simulink library "Lib_EMTAT"  (R2023b)
settings: Solver=VariableStepAuto  StartTime=0.0  StopTime=10.0  RelTol=1e-3
undefined symbols (not defined in the file or in its folder): MWS
libraries: simulink x31, $bdroot x1
(part 1 of 4)
settings Model: Creator=sbianco1  LastModifiedBy=sbianco1
settings SolverCC: AlgebraicLoopSolver=TrustRegion
settings OptimizationCC: BlockReduction=off  DefaultParameterBehavior=Inlined  BufferReuse=off
settings DebuggingCC: UnconnectedInputMsg=warning  UnconnectedOutputMsg=warning  UnconnectedLineMsg=warning
settings ModelReferenceCC: EnableRefExpFcnMdlSchedulingChecks=on
settings RTWCC: DLArmComputeVersion=19.05

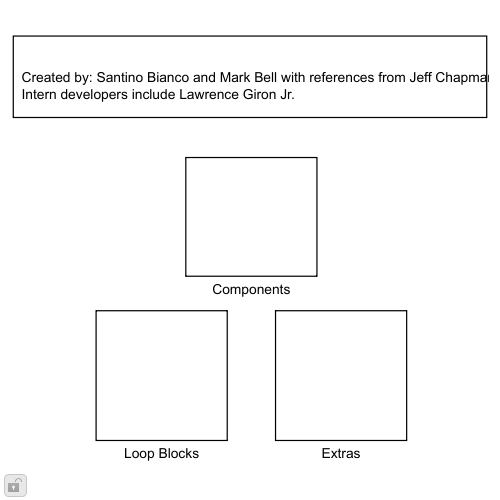
[thumbnail: Simulink's stored preview of the top-level diagram]
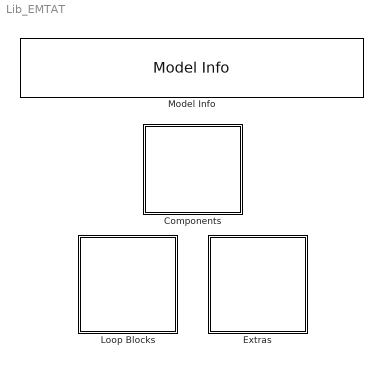
== system Lib_EMTAT ==
  Components : Subsystem
  Extras : Subsystem
  Loop Blocks : Subsystem
  Model Info : simulink/Model-Wide Utilities/Model Info  Frame=on  DisplayStringWithTags=|  HorizontalTextAlignment=Left  LeftAlignmentValue=0.02
      | Created by: Santino Bianco and Mark Bell with references from Jeff Chapman. 
      | Intern developers include Lawrence Giron Jr.

== system Lib_EMTAT/Components ==
  Physics-Based : Subsystem
  Power Flow : Subsystem

== system Lib_EMTAT/Extras ==
  Temperature with Cooling : Subsystem  mask(Component Temperature with Cooling (Ploss)){m=0, Cp=0, COP=0}
      mask prompts: m "m - Mass, lbm"; Cp "Cp - Specific Heat, Btu/(lbm-°F)"; COP "COP=(h*A_s) - Coefficient of Performance, Btu/(hr-°F)"
      mask help: This block calculates the temperature of a component based on the heat generated through power loss (Ploss) and the heat removed by a cooling system modeled as a generic heat exchanger. The block converts a power loss output in units of Watts (Ploss) from an electrical component to a temperature in units of °F (Temp) using the ambient temperature in units of °F (Tamb), and coolant temperature in units of °F (Tin_Cool) as inputs. A mass (m) in units of pound-mass, a specific heat (c_p) in units of Btu/(lbm-°F), and a coefficient of performance (COP) in units of Btu/(hr-°F) must be specified. The component temperature is integrated over time, and thus an initial heat (Q0) in units of Btu must be specified for the integrator block.
      settings: AttributesFormatString=Temperature with Cooling
      mask Help: web('Help_TemperaturewithCooling.html')
      mask DialogControl Container3 Prompt: Physical Parameters

== system Lib_EMTAT/Loop Blocks ==
  Outer Loop Integrator : Subsystem  mask(Outer Loop Integrator){Xo=0}
      mask prompts: Xo "Xo - Initial State Conditions"
      mask help: The Outer Loop Integrator takes in a vector of state variables and integrates each variable using a Continuous Integrator block.
      settings: AttributesFormatString=|
      | Outer Loop Integrator
      | Version: %<LibraryVersion>
      mask DialogControl fsfd Prompt: Parameters
  Outer Loop Time Step Delay : Subsystem  mask(Outer Loop Time Step Delay){Wo=0}
      mask prompts: Wo "Wo - Initial Conditions"
      mask help: The Outer Loop Time Step Delay block takes in a vector of variables and applies a one time step delay to each variable in the vector using a Unit Delay block.
      settings: AttributesFormatString=|
      | OuterLoop Time Step Delay
      | Version: %<LibraryVersion>
      mask DialogControl fsdf Prompt: Parameters

== system Lib_EMTAT/Components/Physics-Based ==

== system Lib_EMTAT/Components/Power Flow ==
  AC-AC Transformer (Efficiency Map) : Subsystem  mask(AC-AC Transformer (Efficiency Map)){X_C_VoltageAC1Vec_M=MWS.I1.Vdc, Y_C_CurrentAC2Vec_M=MWS.I1.Irms, T_C_EffArray_M=MWS.I1.Ploss', K=0.0503, FM=0}
      mask prompts: X_C_VoltageAC1Vec_M "X_C_VoltageAC1Vec_M - Primary AC Line to Neutral RMS Voltage Vector (X-axis)(nx1)"; Y_C_CurrentAC2Vec_M "Y_C_CurrentAC2Vec_M - Secondary RMS Line Current Vector (Y-axis)(mx1)"; T_C_EffArray_M "T_C_EffArray_M - Efficiency Table Values (Ploss = f(Irmsout, Vin)(nxm)"; K "K - Transformer Ratio"; FM "Mode:"
      mask help: This block models an AC/AC transofrmer. The power through the transformer is modified by a user-input efficiency table. The primary side is designated as 1. The secondary side is designated as 2.
      settings: AttributesFormatString=AC-AC Transformer (Efficiency Map)
      mask Help: web(['file:///' which('Help_ACACTransformer_EfficiencyMap.html')])
      mask DialogControl Control3 Prompt: Plot Efficiency Map
      mask DialogControl Control3 Callback:
      | % Plot efficiency map.
      | vals = get_param(gcb,'MaskValues');
      | X = str2num(cell2mat(vals(1)));
      | Y = str2num(cell2mat(vals(2)));
      | Z = str2num(cell2mat(vals(3)));
      | [X,Y] = meshgrid(X,Y);
      | figure('name',[get_param(gcb,'name') ' Efficiency Map'],'numbertitle','off')
      | contour(X,Y,Z,15);
      | xlabel('Voltage In, VDC')
      | ylabel('Line Current Out, A_{rms}')
      | title([get_param(gcb,'name') ' Efficiency Map'])
      | c = colorbar;
      | c.Label.String = 'Efficiency';
      mask DialogControl Container3 Prompt: Failure Modes
      mask DialogControl Control2 Prompt: 1 - Open Circuit, 2 - Degradation
  AC-AC Transformer (Power Loss Map) : Subsystem  mask(AC-AC Transformer (Power Loss Map)){X_C_VoltageAC1Vec_M=MWS.I1.Vdc, Y_C_CurrentAC2Vec_M=MWS.I1.Irms, T_C_PowLossArray_M=MWS.I1.Ploss', K=0.0503, FM=0, Plosslim=0}
      mask prompts: X_C_VoltageAC1Vec_M "X_C_VoltageAC1Vec_M - Primary AC Line to Neutral RMS Voltage Vector (X-axis)(nx1)"; Y_C_CurrentAC2Vec_M "Y_C_CurrentAC2Vec_M - Secondary RMS Line Current Vector (Y-axis)(mx1)"; T_C_PowLossArray_M "T_C_PowLossArray_M - Power Loss Table Values (Ploss = f(Irmsout, Vin)(nxm)"; K "K - Transformer Ratio"; FM "Mode:"; Plosslim "Plosslim - Power Loss Limit, W"
      mask help: This block models an AC/AC transofrmer. The power through the transformer is modified by a user-input power loss table. The primary side is designated as 1. The secondary side is designated as 2.
      settings: AttributesFormatString=AC-AC Transformer (Power Loss Map)
      mask Help: web(['file:///' which('Help_ACACTransformer_PowerLossMap.html')])
      mask DialogControl Control3 Prompt: Plot Power Loss Map
      mask DialogControl Control3 Callback:
      | % Plot efficiency map.
      | vals = get_param(gcb,'MaskValues');
      | X = str2num(cell2mat(vals(1)));
      | Y = str2num(cell2mat(vals(2)));
      | Z = str2num(cell2mat(vals(3)));
      | [X,Y] = meshgrid(X,Y);
      | figure('name',[get_param(gcb,'name') ' Power Loss Map'],'numbertitle','off')
      | contour(X,Y,Z,15);
      | xlabel('Voltage In, VDC')
      | ylabel('Line Current Out, A_{rms}')
      | title([get_param(gcb,'name') ' Power Loss Map'])
      | c = colorbar;
      | c.Label.String = 'Power Loss, W';
      mask DialogControl Container3 Prompt: Failure Modes
      mask DialogControl Control2 Prompt: 1 - Open Circuit, 2 - Degradation
  AC-DC Rectifier (Efficiency Map) : Subsystem  mask(AC - DC Rectifier (Efficiency Map)){X_C_VoltageInVec_M=[0 1000], Y_C_RMSCurrentOutVec_M=[0 1000], T_C_EffArray_M=ones(2), T_C_PFArray_M=ones(2), FM=0}
      mask prompts: X_C_VoltageInVec_M "X_C_VoltageInVec_M - DC Voltage Vector, V (m x 1)"; Y_C_RMSCurrentOutVec_M "Y_C_RMSCurrentOutVec_M - RMS Line Current Vector, Arms (p x 1)"; T_C_EffArray_M "T_C_EffArray_M - Efficiency Table Values, W (m x p)"; T_C_PFArray_M "T_C_PFArray_M - Power Factor Table Values, W (m x p)"; FM "Mode:"
      mask help: This block models an inverter/rectifier for use as a power source. The power through the inverter/rectifier is modified by a user-input efficiency and power factor tables.
      settings: AttributesFormatString=AC-DC Rectifier (Efficiency Map)
      mask Help: web(['file:///' which('Help_AC_DCRectifier_EfficiencyMap.html')])
      mask DialogControl Control2 Prompt: Plot Efficiency and Power Factor Maps
      mask DialogControl Control2 Callback:
      | % Plot efficiency map.
      | vals = get_param(gcb,'MaskValues');
      | X = str2num(cell2mat(vals(1)));
      | Y = str2num(cell2mat(vals(2)));
      | Z = str2num(cell2mat(vals(3)));
      | ZZ = str2num(cell2mat(vals(4)));
      | [X,Y] = meshgrid(X,Y);
      | figure('name',[get_param(gcb,'name') ' Efficiency and Power Factor Maps'],'numbertitle','off')
      | subplot(2,1,1)
      | contour(X,Y,Z,15);
      | xlabel('Voltage In, VDC')
      | ylabel('Line Current Out, A_{rms}')
      | title([get_param(gcb,'name') ' Efficiency Map'])
      | c = colorbar;
      | c.Label.String = 'Efficiency';
      | 
      | subplot(2,1,2)
      | contour(X,Y,ZZ,15);
      | xlabel('Voltage In, VDC')
      | ylabel('Line Current Out, A_{rms}')
      | title([get_param(gcb,'name') ' Power Factor Map'])
      | c = colorbar;
      | c.Label.String = 'Power Factor';
      mask DialogControl Container3 Prompt: Failure Modes
      mask DialogControl Control3 Prompt: 1 - Open Circuit, 2 - Efficiency Scalar
  AC-DC Rectifier (Power Loss Map) : Subsystem  mask(AC-DC Rectifier (Power Loss Map)){X_C_VoltageInVec_M=[0 1000], Y_C_RMSCurrentOutVec_M=[0 1000], T_C_PowLossArray_M=0*ones(2), T_C_PFArray_M=ones(2), FM=0, Plosslim=0}
      mask prompts: X_C_VoltageInVec_M "X_C_VoltageInVec_M - DC Voltage Vector, V (m x 1)"; Y_C_RMSCurrentOutVec_M "Y_C_RMSCurrentOutVec_M - RMS Line Current Vector, Arms (p x 1)"; T_C_PowLossArray_M "T_C_PowLossArray_M - Power Loss Table Values, W (m x p)"; T_C_PFArray_M "T_C_PFArray_M - Power Loss Table Values, W (m x p)"; FM "Mode:"; Plosslim "Plosslim - Power Loss Limit, W"
      mask help: This block models an inverter/rectifier for use as a power source. The power through the inverter/rectifier is modified by a user-input power loss and power factor tables.
      settings: AttributesFormatString=AC-DC Rectifier (Power Loss Map)
      mask Help: web(['file:///' which('Help_AC_DCRectifier_PowerLossMap.html')])
      mask DialogControl Control2 Prompt: Plot Power Loss and Power Factor Maps
      mask DialogControl Control2 Callback:
      | % Plot efficiency map.
      | vals = get_param(gcb,'MaskValues');
      | X = str2num(cell2mat(vals(1)));
      | Y = str2num(cell2mat(vals(2)));
      | Z = str2num(cell2mat(vals(3)));
      | ZZ = str2num(cell2mat(vals(4)));
      | [X,Y] = meshgrid(X,Y);
      | figure('name',[get_param(gcb,'name') ' Power Loss and Power Factor Maps'],'numbertitle','off')
      | subplot(2,1,1)
      | contour(X,Y,Z,15);
      | xlabel('Voltage In, VDC')
      | ylabel('Line Current Out, A_{rms}')
      | title([get_param(gcb,'name') ' Power Loss Map'])
      | c = colorbar;
      | c.Label.String = 'Power Loss, W';
      | 
      | subplot(2,1,2)
      | contour(X,Y,ZZ,15);
      | xlabel('Voltage In, VDC')
      | ylabel('Line Current Out, A_{rms}')
      | title([get_param(gcb,'name') ' Power Factor Map'])
      | c = colorbar;
      | c.Label.String = 'Power Factor';
      mask DialogControl Container3 Prompt: Failure Modes
      mask DialogControl Control3 Prompt: 1 - Open Circuit, 2 - Power Scalar
  Battery : Subsystem  mask(Generic Battery Model){ESR=0.005, Vcharge_vec=[3.60022000000000  3.47014090756723  3.40534522081438  3.36797345615108  3.34637300833001  3.33384164719904  3.32652442405484  3.32220404518678  3.31960513667983  3.31799408159663  3.31694886010866  3.31622666940565  3.31568778312557  3.31525175779256  3.31487224411964  3.31452249917241  3.31418705328483  3.31385691696240  3.31352682385014  3.31319364476023  3.31285547523761  3.31251111050485  3.31215974319668  3.31180078921639  3.31143378726315  3.31105834070993  3.31067408381608  3.31028066191027  3.30987771958033  3.30946489343758  3.30904180747880  3.30860806990567  3.30816327074273  3.30770697987113  3.30723874525401  3.30675809122011  3.30626451672401  3.30575749353022  3.30523646428523  3.30470084044935  3.30415000006513  3.30358328534007  3.30300000002157  3.30239940654061  3.30178072289873  3.30114311927020  3.30048571428812  3.29980757097933  3.29910769230854  3.29838501628717  3.29763841059637  3.29686666666691  3.29606849315088  3.29524250871097  3.29438723404271  3.29350108303264  3.29258235294130  3.29162921348325  3.29063969465657  3.28961167315181  3.28854285714290  3.28743076923078  3.28627272727272  3.28506582278477  3.28380689655166  3.28249251101312  3.28111891891878  3.27968202764960  3.27817735849035  3.27659999999974  3.27494455445513  3.27320507614176  3.27137499999957  3.26944705882304  3.26741318681262  3.26526440677901  3.26299069767368  3.26058083832252  3.25802222222128  3.25530063694161  3.25239999999879  3.24930204081497  3.24598591549143  3.24242773722455  3.23859999999805  3.23447086613954  3.23000327868604  3.22515384615104  3.21987142856824  3.21409532709918  3.20775294117234  3.20075670102620  3.19299999999457  3.18435172413165  3.17464878048051  3.16368571427719  3.15119999998996  3.13685074625673  3.12018709675987  3.10059999998259  3.07724615382467  3.04892340422834  3.01385714282250  2.96931351346777  2.91084999993737  2.83073333324329  2.71419999986125  2.52911764682123  2.18979999951267  1.36574285567986], Vdischarge_vec=[3.60022000000000  3.47014090756723  3.40534522081438  3.36797345615108  3.34637300833001  3.33384164719904  3.32652442405484  3.32220404518678  3.31960513667983  3.31799408159663  3.31694886010866  3.31622666940565  3.31568778312557  3.31525175779256  3.31487224411964  3.31452249917241  3.31418705328483  3.31385691696240  3.31352682385014  3.31319364476023  3.31285547523761  3.31251111050485  3.31215974319668  3.31180078921639  3.31143378726315  3.31105834070993  3.31067408381608  3.31028066191027  3.30987771958033  3.30946489343758  3.30904180747880  3.30860806990567  3.30816327074273  3.30770697987113  3.30723874525401  3.30675809122011  3.30626451672401  3.30575749353022  3.30523646428523  3.30470084044935  3.30415000006513  3.30358328534007  3.30300000002157  3.30239940654061  3.30178072289873  3.30114311927020  3.30048571428812  3.29980757097933  3.29910769230854  3.29838501628717  3.29763841059637  3.29686666666691  3.29606849315088  3.29524250871097  3.29438723404271  3.29350108303264  3.29258235294130  3.29162921348325  3.29063969465657  3.28961167315181  3.28854285714290  3.28743076923078  3.28627272727272  3.28506582278477  3.28380689655166  3.28249251101312  3.28111891891878  3.27968202764960  3.27817735849035  3.27659999999974  3.27494455445513  3.27320507614176  3.27137499999957  3.26944705882304  3.26741318681262  3.26526440677901  3.26299069767368  3.26058083832252  3.25802222222128  3.25530063694161  3.25239999999879  3.24930204081497  3.24598591549143  3.24242773722455  3.23859999999805  3.23447086613954  3.23000327868604  3.22515384615104  3.21987142856824  3.21409532709918  3.20775294117234  3.20075670102620  3.19299999999457  3.18435172413165  3.17464878048051  3.16368571427719  3.15119999998996  3.13685074625673  3.12018709675987  3.10059999998259  3.07724615382467  3.04892340422834  3.01385714282250  2.96931351346777  2.91084999993737  2.83073333324329  2.71419999986125  2.52911764682123  2.18979999951267  1.36574285567986], It_vec=[0  0.0209908023779841  0.0419816047559682  0.0629724071339524  0.0839632095119365  0.104954011889921  0.125944814267905  0.146935616645889  0.167926419023873  0.188917221401857  0.209908023779841  0.230898826157825  0.251889628535809  0.272880430913794  0.293871233291778  0.314862035669762  0.335852838047746  0.356843640425730  0.377834442803714  0.398825245181698  0.419816047559682  0.440806849937666  0.461797652315651  0.482788454693635  0.503779257071619  0.524770059449603  0.545760861827587  0.566751664205571  0.587742466583555  0.608733268961539  0.629724071339524  0.650714873717508  0.671705676095492  0.692696478473476  0.713687280851460  0.734678083229444  0.755668885607428  0.776659687985412  0.797650490363396  0.818641292741380  0.839632095119365  0.860622897497349  0.881613699875333  0.902604502253317  0.923595304631301  0.944586107009285  0.965576909387269  0.986567711765253  1.00755851414324  1.02854931652122  1.04954011889921  1.07053092127719  1.09152172365517  1.11251252603316  1.13350332841114  1.15449413078913  1.17548493316711  1.19647573554509  1.21746653792308  1.23845734030106  1.25944814267905  1.28043894505703  1.30142974743502  1.32242054981300  1.34341135219098  1.36440215456897  1.38539295694695  1.40638375932494  1.42737456170292  1.44836536408090  1.46935616645889  1.49034696883687  1.51133777121486  1.53232857359284  1.55331937597082  1.57431017834881  1.59530098072679  1.61629178310478  1.63728258548276  1.65827338786075  1.67926419023873  1.70025499261671  1.72124579499470  1.74223659737268  1.76322739975067  1.78421820212865  1.80520900450663  1.82619980688462  1.84719060926260  1.86818141164059  1.88917221401857  1.91016301639655  1.93115381877454  1.95214462115252  1.97313542353051  1.99412622590849  2.01511702828648  2.03610783066446  2.05709863304244  2.07808943542043  2.09908023779841  2.12007104017640  2.14106184255438  2.16205264493236  2.18304344731035  2.20403424968833  2.22502505206632  2.24601585444430  2.26700665682228  2.28799745920027]}
      mask prompts: ESR "Equivalent Series  Resistance - ESR (Ohm)"; Vcharge_vec "Battery Voltage Charge Curve (V)"; Vdischarge_vec "Battery Voltage Discharge Curve (V)"; It_vec "Capacity Table (Depth of Discharge) (Ah)"
      mask help: This is a block that models the voltage response of a generic battery based on the current demand. The block parameters are the internal resistance and the charge/discharge curves, which are defined as state of charge (SOC) vs. Voltage. Separate charge and discharge curves can be defined to allow for battery charge hysteresis.
      mask init:
      | BN = gcb;
      settings: AttributesFormatString=Battery
      mask Help: web(['file:///' which('Help_Battery.html')])
      mask DialogControl DescTextVar Prompt: Battery Model
  Cable : Subsystem  mask(Cable){R=0.2}
      mask prompts: R "R - Resistance, Ohm"
      mask help: This block models a cable with resistive effects.
      settings: AttributesFormatString=Cable
      mask Help: web(['file:///' which('Help_Cable.html')])
      mask DialogControl Container3 Prompt: Failure Modes
      mask DialogControl Control2 Prompt: Mode: Open Circuit
  Current Distribution : Subsystem  mask(Current Distribution){}
      settings: AttributesFormatString=Current Distribution
      mask Help: web(['file:///' which('Help_CurrentDistribution.html')])
  Current Junction : Subsystem  mask(Current Junction){Nb=1}
      mask prompts: Nb "Nb - # of branches"
      mask help: This block adds a vector of input currents (I).
      settings: AttributesFormatString=Current Junction
      mask Help: web(['file:///' which('Help_CurrentJunction.html')])
      mask DialogControl Control2 Prompt: Note: There is no limit to the number of multiplexed currents.
      mask DialogControl Container2 Prompt: Parameters
  DC-AC Inverter (Efficiency Map) : Subsystem  mask(DC-AC Inverter (Efficiency Map)){X_C_VoltageInVec_M=[0 1000], Y_C_RMSCurrentOutVec_M=[0 1000], T_C_EffArray_M=ones(2), T_C_PFArray_M=ones(2), K_e=0.0503, FM=0}
      mask prompts: X_C_VoltageInVec_M "X_C_VoltageInVec_M - DC Voltage Vector (X-axis)(nx1)"; Y_C_RMSCurrentOutVec_M "Y_C_RMSCurrentOutVec_M - RMS Line Current Vector (Y-axis)(mx1)"; T_C_EffArray_M "T_C_EffArray_M - Efficiency Table Values (Eff = f(Irmsout, Vin)(nxm)"; T_C_PFArray_M "T_C_PFArray_M - Power Factor Table Values (Eff = f(Irmsout, Vin)(nxm)"; K_e "K_e - Back EMF Constant, V_LL_peak/RPM"; FM "Mode:"
      mask help:
      | This block models an inverter/rectifier for use as a power sink. The power through the inverter/rectifier is modified by a user-input efficiency and power factor tables
      | .
      settings: AttributesFormatString=DC-AC Inverter (Efficiency Map)
      mask Help: web(['file:///' which('Help_DC_ACInverter_EfficiencyMap.html')])
      mask DialogControl Control3 Prompt: Plot Efficiency and Power Factor Maps
      mask DialogControl Control3 Callback:
      | % Plot efficiency map.
      | vals = get_param(gcb,'MaskValues');
      | X = str2num(cell2mat(vals(1)));
      | Y = str2num(cell2mat(vals(2)));
      | Z = str2num(cell2mat(vals(3)));
      | ZZ = str2num(cell2mat(vals(4)));
      | 
      | [X,Y] = meshgrid(X,Y);
      | figure('name',[get_param(gcb,'name') ' Efficiency and Power Factor Map'],'numbertitle','off')
      | subplot(2,1,1)
      | contour(X,Y,Z,15);
      | xlabel('Voltage In, VDC')
      | ylabel('Line Current Out, A_{rms}')
      | title([get_param(gcb,'name') ' Efficiency Map'])
      | c = colorbar;
      | c.Label.String = 'Efficiency';
      | 
      | subplot(2,1,2)
      | contour(X,Y,ZZ,15);
      | xlabel('Voltage In, VDC')
      | ylabel('Line Current Out, A_{rms}')
      | title([get_param(gcb,'name') ' Power Factor Map'])
      | c = colorbar;
      | c.Label.String = 'Power Factor';
      mask DialogControl Container3 Prompt: Failure Modes
      mask DialogControl Control2 Prompt: 1 - Open Circuit, 2 - Efficiency Scalar
  DC-AC Inverter (Power Loss Map) : Subsystem  mask(DC-AC Inverter (Power Loss Map)){X_C_VoltageInVec_M=[0 1000], Y_C_RMSCurrentOutVec_M=[0 1000], T_C_PowLossArray_M=zeros(2), T_C_PFArray_M=ones(2), K_e=0.0503, FM=0, Plosslim=0}
      mask prompts: X_C_VoltageInVec_M "X_C_VoltageInVec_M - DC Voltage Vector (X-axis)(nx1)"; Y_C_RMSCurrentOutVec_M "Y_C_RMSCurrentOutVec_M - RMS Line Current Vector (Y-axis)(mx1)"; T_C_PowLossArray_M "T_C_PowLossArray_M - Power Loss Table Values (Ploss = f(Irmsout, Vin)(nxm)"; T_C_PFArray_M "T_C_PFArray_M - Power Factor Table Values (Ploss = f(Irmsout, Vin)(nxm)"; K_e "K_e - Back EMF Constant, V_LL_peak/RPM"; FM "Mode:"; Plosslim "Plosslim - Power Loss Limit, W"
      mask help: This block models an inverter/rectifier for use as a power sink. The power through the inverter/rectifier is modified by a user-input power loss and power factor tables.
      settings: AttributesFormatString=DC-AC Inverter (Power Loss Map)
      mask Help: web(['file:///' which('Help_DC_ACInverter_PowerLossMap.html')])
      mask DialogControl Control3 Prompt: Plot Power Loss and Power Factor Maps
      mask DialogControl Control3 Callback:
      | % Plot efficiency map.
      | vals = get_param(gcb,'MaskValues');
      | X = str2num(cell2mat(vals(1)));
      | Y = str2num(cell2mat(vals(2)));
      | Z = str2num(cell2mat(vals(3)));
      | ZZ = str2num(cell2mat(vals(4)));
      | [X,Y] = meshgrid(X,Y);
      | figure('name',[get_param(gcb,'name') ' Power Loss and Power Factor Map'],'numbertitle','off')
      | subplot(2,1,1)
      | contour(X,Y,Z,15);
      | xlabel('Voltage In, VDC')
      | ylabel('Line Current Out, A_{rms}')
      | title([get_param(gcb,'name') ' Power Loss Map'])
      | c = colorbar;
      | c.Label.String = 'Power Loss, W';
      | 
      | subplot(2,1,2)
      | contour(X,Y,ZZ,15);
      | xlabel('Voltage In, VDC')
      | ylabel('Line Current Out, A_{rms}')
      | title([get_param(gcb,'name') ' Power Factor Map'])
      | c = colorbar;
      | c.Label.String = 'Power Factor';
      mask DialogControl Container3 Prompt: Failure Modes
      mask DialogControl Control2 Prompt: 1 - Open Circuit, 2 - Power Loss Scalar
  DC-DC Converter (Efficiency Map) (Regulate Output Voltage) : Subsystem  mask(DC-DC Converter (Efficiency Map) (Regulate Output Voltage)){X_Vin_VoltageVec_M=[0 100 1000 5000], Y_Iout_CurrentVec_M=[0 10 100 150], T_C_EffArray_M=0.98*ones(4,4), FM=0}
      mask prompts: X_Vin_VoltageVec_M "X_Vin_VoltageVec_M - Efficiency Table Voltage In Vector (X-axis)(nx1)"; Y_Iout_CurrentVec_M "Y_Iout_CurrentVec_M - Efficiency Table Current Out Vector (Y-axis)(mx1)"; T_C_EffArray_M "T_C_EffArray_M - Efficiency Table Values (Eff = f(i, V)(nxm)"; FM "Mode:"
      mask help: This block models the power flow through a DC-DC converter using a user specified efficiency table. The output voltage (Vout) can also be set using variable Vset.
      settings: AttributesFormatString=|
      | DC-DC Converter
      | (Efficiency Map)
      | (Regulate Output Voltage)
      mask Help: web(['file:///' which('Help_DCDCConverter_EfficiencyMap_RegulateOutputVoltage.html')])
      mask DialogControl Control3 Prompt: Plot Efficiency Map
      mask DialogControl Control3 Callback:
      | % Plot power loss map.
      | vals = get_param(gcb,'MaskValues');
      | X = str2num(cell2mat(vals(1)));
      | Y = str2num(cell2mat(vals(2)));
      | Z = str2num(cell2mat(vals(3)));
      | [X,Y] = meshgrid(X,Y);
      | figure('name',[get_param(gcb,'name') ' Efficiency Map'],'numbertitle','off')
      | contour(X,Y,Z,15);
      | xlabel('Voltage In, VDC')
      | ylabel('Current Out, ADC')
      | title([get_param(gcb,'name') ' Efficiency Map'])
      | c = colorbar;
      | c.Label.String = 'Efficiency';
      mask DialogControl Container3 Prompt: Failure Modes
      mask DialogControl Control2 Prompt: 1 - Open Circuit, 2 - Degradation
  DC-DC Converter (Efficiency Map) (Set Output Voltage) : Subsystem  mask(DC-DC Converter (Efficiency Map) (Set Output Voltage)){X_Vin_VoltageVec_M=[0 100 1000 5000], Y_Iout_CurrentVec_M=[0 10 100 150], T_C_EffArray_M=0.98*ones(4,4), FM=0}
      mask prompts: X_Vin_VoltageVec_M "X_Vin_VoltageVec_M - Efficiency Table Voltage In Vector, V (m x 1)"; Y_Iout_CurrentVec_M "Y_Iout_CurrentVec_M - Efficiency Table Current Out Vector, A (p x 1)"; T_C_EffArray_M "T_C_EffArray_M - Efficiency Table Values, W (m x p)"; FM "Mode:"
      mask help: This block models the power flow through a DC-DC converter using a user specified efficiency table. The output voltage (V_2) can be set using variable V*.
      settings: AttributesFormatString=|
      | DC-DC Converter
      | (Efficiency Map)
      | (Set Output Voltage)
      mask Help: web(['file:///' which('Help_DCDCConverter_EfficiencyMap_SetOutputVoltage.html')])
      mask DialogControl Control3 Prompt: Plot Efficiency Map
      mask DialogControl Control3 Callback:
      | % Plot power loss map.
      | vals = get_param(gcb,'MaskValues');
      | X = str2num(cell2mat(vals(1)));
      | Y = str2num(cell2mat(vals(2)));
      | Z = str2num(cell2mat(vals(3)));
      | [X,Y] = meshgrid(X,Y);
      | figure('name',[get_param(gcb,'name') ' Efficiency Map'],'numbertitle','off')
      | contour(X,Y,Z,15);
      | xlabel('Voltage In, VDC')
      | ylabel('Current Out, ADC')
      | title([get_param(gcb,'name') ' Efficiency Map'])
      | c = colorbar;
      | c.Label.String = 'Efficiency';
      mask DialogControl Container3 Prompt: Failure Modes
      mask DialogControl Control2 Prompt: 1 - Open Circuit, 2 - Degradation
  DC-DC Converter (Power Loss Map) (Regulate Output Voltage) : Subsystem  mask(DC-DC Converter (Power Loss Map) (Regulate Output Voltage)){X_Vin_VoltageVec_M=[0 100 1000 5000], Y_Iout_CurrentVec_M=[0 10 100 150], T_C_PlossArray_M=0.98*ones(4,4), FM=0, Plosslim=0}
      mask prompts: X_Vin_VoltageVec_M "X_Vin_VoltageVec_M - Efficiency Table Voltage In Vector (X-axis)(nx1)"; Y_Iout_CurrentVec_M "Y_Iout_CurrentVec_M - Efficiency Table Current Out Vector (Y-axis)(mx1)"; T_C_PlossArray_M "T_C_PlossArray_M - Power Loss Table Values (Eff = f(i, V)(nxm)"; FM "Mode:"; Plosslim "Plosslim - Power Loss Limit, W"
      mask help: This block models the power flow through a DC-DC converter using a user specified power loss table. The output voltage (Vout) can also be set using variable Vset.
      settings: AttributesFormatString=|
      | DC-DC Converter
      | (Power Loss Map)
      | (Regulate Output Voltage)
      mask Help: web(['file:///' which('Help_DCDCConverter_PowerLossMap_RegulateOutputVoltage.html')])
      mask DialogControl Control3 Prompt: Plot Power Loss Map
      mask DialogControl Control3 Callback:
      | % Plot power loss map.
      | vals = get_param(gcb,'MaskValues');
      | X = str2num(cell2mat(vals(1)));
      | Y = str2num(cell2mat(vals(2)));
      | Z = str2num(cell2mat(vals(3)));
      | [X,Y] = meshgrid(X,Y);
      | figure('name',[get_param(gcb,'name') ' Power Loss Map'],'numbertitle','off')
      | contour(X,Y,Z,15);
      | xlabel('Voltage In, VDC')
      | ylabel('Current Out, ADC')
      | title([get_param(gcb,'name') ' Power Loss Map'])
      | c = colorbar;
      | c.Label.String = 'Power loss, W';
      mask DialogControl Container3 Prompt: Failure Modes
      mask DialogControl Control2 Prompt: 1 - Open Circuit, 2 - Degradation
  DC-DC Converter (Power Loss Map) (Set Output Voltage) : Subsystem  mask(DC-DC Converter (Power Loss Map) (Set Output Voltage)){X_Vin_VoltageVec_M=[0 100 1000 5000], Y_Iout_CurrentVec_M=[0 10 100 150], T_C_PlossArray_M=0.98*ones(4,4), FM=0, Plosslim=0}
      mask prompts: X_Vin_VoltageVec_M "X_Vin_VoltageVec_M - Efficiency Table Voltage In Vector, V (m x 1)"; Y_Iout_CurrentVec_M "Y_Iout_CurrentVec_M - Efficiency Table Current Out Vector, A (p x 1)"; T_C_PlossArray_M "T_C_PlossArray_M - Power Loss Table Values, W (m x p)"; FM "Mode:"; Plosslim "Plosslim - Power Loss Limit, W"
      mask help: This block models the power flow through a DC-DC converter using a user specified power loss table. The output voltage (V_2) can be set using variable V*.
      settings: AttributesFormatString=|
      | DC-DC Converter
      | (Power Loss Map)
      | (Set Output Voltage)
      mask Help: web(['file:///' which('Help_DCDCConverter_PowerLossMap_SetOutputVoltage.html')])
      mask DialogControl Control3 Prompt: Plot Power Loss Map
      mask DialogControl Control3 Callback:
      | % Plot power loss map.
      | vals = get_param(gcb,'MaskValues');
      | X = str2num(cell2mat(vals(1)));
      | Y = str2num(cell2mat(vals(2)));
      | Z = str2num(cell2mat(vals(3)));
      | [X,Y] = meshgrid(X,Y);
      | figure('name',[get_param(gcb,'name') ' Power Loss Map'],'numbertitle','off')
      | contour(X,Y,Z,15);
      | xlabel('Voltage In, VDC')
      | ylabel('Current Out, ADC')
      | title([get_param(gcb,'name') ' Power Loss Map'])
      | c = colorbar;
      | c.Label.String = 'Power loss, W';
      mask DialogControl Container3 Prompt: Failure Modes
      mask DialogControl Control2 Prompt: 1 - Open Circuit, 2 - Degradation
  Electrical Bus : Subsystem  mask(Bus){C=6e-3, Nb=1}
      mask prompts: C "C - Capacitance, F"; Nb "Nb - # of branches"
      mask help: This block represents an electrical bus with capacitance effects.
      settings: AttributesFormatString=Electrical Bus
      mask Help: web(['file:///' which('Help_ElectricalBus.html')])
  Mechanical Shaft : Subsystem  mask(Mechanical Shaft){J=0.01, B=0.001}
      mask prompts: J "J - Inertia, lb-ft-s^2"; B "B - Damping, lb-ft-s"
      mask help: This block models a mechanical shaft with inertial and viscous damping effects.
      settings: AttributesFormatString=Mechanical Shaft
      mask Help: web(['file:///' which('Help_MechanicalShaft.html')])
      mask DialogControl Container3 Prompt: Failure Mode
      mask DialogControl Control2 Prompt: Mode: Shaft Break
  Power Supply (Set Voltage) : Subsystem  mask(Power Supply (Set Voltage)){Nb=0}
      mask prompts: Nb "Nb - # of branches"
      mask help: This block models a power supply that uses Vset to set, not regulate, the bus voltage based on a vector of current demands (Idmd).
      settings: AttributesFormatString=|
      | Power Supply
      | (Set Voltage)
      mask Help: web(['file:///' which('Help_PowerSupply_SetVoltage.html')])
      mask DialogControl Container2 Prompt: Parameters
  Resistive Load Bank : Subsystem  ClipboardFcn=|  mask(Resistive Load Bank){}
      | Active Resistor
      | Version: %<LibraryVersion>
      mask help: This block changes its resistance (R) based on a power command (Pset) to produce a current demand (Iin).
      settings: AttributesFormatString=Resistive Load Bank
      mask Help: web(['file:///' which('Help_ResistiveLoadBank.html')])
      mask DialogControl Container2 Prompt: Failure Modes
      mask DialogControl Control2 Prompt: Mode: Open Circuit
  Supercapacitor : Subsystem  mask(Supercapacitor){C=130, ESR=0.02, TSE=69, BlkNm=double(gcb)}
      mask prompts: C "C - Capacitance, F"; ESR "ESR - Equivilent Series Resistance, Ohm"; TSE "TSE - Max Stored Energy, W-h"; BlkNm "Block Name"
      mask help: This block models a capacitor with equivilent series resistive (ESR) effects.
      mask init:
      | BN = gcb;
      settings: AttributesFormatString=Supercapacitor
      mask Help: web(['file:///' which('Help_Supercapacitor.html')])
  Three Phase Electric Machine (Sink) : Subsystem  mask(Three Phase Electric Machine (Sink)){X_C_SpeedVec_M=[0 8000], Y_C_TorqueVec_M=[0 300], T_C_EffArray_M=[0.97 0.95; 0.93 0.94], T_C_PFArray_M=[1 1;1 1], FM=0}
      mask prompts: X_C_SpeedVec_M "X_C_SpeedVec_M - Efficiency Table Speed Vector (nx1)"; Y_C_TorqueVec_M "Y_C_TorqueVec_M - Efficiency Table Torque Vector (mx1)"; T_C_EffArray_M "T_C_EffArray_M - Efficiency Table Values (nxm)"; T_C_PFArray_M "T_C_PFArray_M - Power Factor Table Values (nxm)"; FM "Mode:"
      mask help: This block models an three phase motor/generator for use as a power sink. The power through the motor/generator is modified by a user-input efficiency and power factor tables.
      settings: AttributesFormatString=|
      | Three Phase Electric Machine
      | (Sink)
      mask Help: web(['file:///' which('Help_ThreePhaseElectricMachineSink.html')])
      mask DialogControl Container2 Prompt: Parameters
      mask DialogControl Plot Prompt: Plot Efficiency and Power Factor Maps
      mask DialogControl Plot Callback:
      | % Plot efficiency map.
      | vals = get_param(gcb,'MaskValues');
      | X = str2num(cell2mat(vals(1)));
      | Y = str2num(cell2mat(vals(2)));
      | Z = str2num(cell2mat(vals(3)));
      | ZZ = str2num(cell2mat(vals(4)));
      | [X,Y] = meshgrid(X,Y);
      | 
      | figure('name',[get_param(gcb,'name') ' Efficiency and Power Factor Map'],'numbertitle','off')
      | subplot(2,1,1)
      | contour(X,Y,Z,15);
      | xlabel('Speed, RPM')
      | ylabel('Torque, lbf-ft')
      | title([get_param(gcb,'name') ' Efficiency Map'])
      | c = colorbar;
      | c.Label.String = 'Efficiency';
      | 
      | subplot(2,1,2)
      | contour(X,Y,ZZ,15);
      | xlabel('Speed, RPM')
      | ylabel('Torque, lbf-ft')
      | title([get_param(gcb,'name') ' Power Factor Map'])
      | c = colorbar;
      | c.Label.String = 'Power Factor';
      mask DialogControl Container3 Prompt: Failure Modes
      mask DialogControl Control3 Prompt: 1 - Open Circuit, 2 - Efficiency Scaling
  Three Phase Electric Machine (Source) : Subsystem  mask(Three Phase Electric Machine (Source)){X_C_SpeedVec_M=[0 10000], Y_C_TorqueVec_M=[0 500], T_C_EffArray_M=0.9*ones(2), T_C_PFArray_M=[1,1;1,1], Ke=0.05, FM=0}
      mask prompts: X_C_SpeedVec_M "X_C_SpeedVec_M - Efficiency Table Speed Vector (X-axis)(nx1)"; Y_C_TorqueVec_M "Y_C_TorqueVec_M - Efficiency Table Torque Vector (Y-axis)(mx1)"; T_C_EffArray_M "T_C_EffArray_M - Efficiency Table Values (nxm)"; T_C_PFArray_M "T_C_PFArray_M - Power Fector Table Values (nxm)"; Ke "Ke - Back EMF Constant, V_LL_peak/RPM"; FM "Mode:"
      mask help: This block models an motor/generator for use as a power source. The power through the motor/generator is modified by a user-input efficiency and power factor tables.
      settings: AttributesFormatString=|
      | Three Phase Electric Machine
      | (Source)
      mask Help: web(['file:///' which('Help_ThreePhaseElectricMachineSource.html')])
      mask DialogControl Control2 Prompt: Plot Efficiency and Power Loss Maps
      mask DialogControl Control2 Callback:
      | % Plot efficiency map.
      | vals = get_param(gcb,'MaskValues');
      | X = str2num(cell2mat(vals(1)));
      | Y = str2num(cell2mat(vals(2)));
      | Z = str2num(cell2mat(vals(3)));
      | ZZ = str2num(cell2mat(vals(4)));
      | [X,Y] = meshgrid(X,Y);
      | 
      | figure('name',[get_param(gcb,'name') ' Efficiency and Power Factor Map'],'numbertitle','off')
      | subplot(2,1,1)
      | contour(X,Y,Z,15);
      | xlabel('Speed, RPM')
      | ylabel('Torque, lbf-ft')
      | title([get_param(gcb,'name') ' Efficiency Map'])
      | c = colorbar;
      | c.Label.String = 'Efficiency';
      | 
      | subplot(2,1,2)
      | contour(X,Y,ZZ,15);
      | xlabel('Speed, RPM')
      | ylabel('Torque, lbf-ft')
      | title([get_param(gcb,'name') ' Power Factor Map'])
      | c = colorbar;
      | c.Label.String = 'Power Factor';
      mask DialogControl Container3 Prompt: Failure Modes
      mask DialogControl Control3 Prompt: 1 - Open Circuit, 2 - Efficiency Scalar

== system Lib_EMTAT/Extras/Temperature with Cooling ==
  "Ploss, W" : Inport
  "Tamb, degF" : Inport  Port=2
  "Tcool, degF" : Inport  Port=3
  "T(t-1), degF" : Inport  Port=4
  "Q, J" : Inport  Port=5
  BTU/hr to Watts : Gain  Gain=0.29307
  Coefficient of Performance (Btu/(hr-°F)) : Constant  Value=COP
  Divide : Product  Inputs=*//
  Joules to BTU : Gain  Gain=0.000947817
  Mass (lbm) : Constant  Value=m
  Multiply1 : Product  Inputs=**
  Specific Heat (Btu/(lbm-°F)) : Constant  Value=Cp
  Subtract : Sum  Inputs=-+
  Subtract2 : Sum  Inputs=+-
  Sum : Sum  Inputs=|++
  "T, degF" : Outport
  "T(t), degF" : Outport  Port=2
  "Qdot, W" : Outport  Port=3
  wires:
  "Tamb, degF"/1 -> Sum/2
  Joules to BTU/1 -> Divide/1
  Specific Heat (Btu/(lbm-°F))/1 -> Divide/3
  Coefficient of Performance (Btu/(hr-°F))/1 -> Multiply1/2
  "Q, J"/1 -> Joules to BTU/1
  "Tcool, degF"/1 -> Subtract2/2
  Subtract2/1 -> Multiply1/1
  Sum/1 -> "T(t), degF"/1, "T, degF"/1
  "T(t-1), degF"/1 -> Subtract2/1
  "Ploss, W"/1 -> Subtract/2
  Mass (lbm)/1 -> Divide/2
  Divide/1 -> Sum/1
  Subtract/1 -> "Qdot, W"/1
  Multiply1/1 -> BTU/hr to Watts/1
  BTU/hr to Watts/1 -> Subtract/1

== system Lib_EMTAT/Loop Blocks/Outer Loop Integrator ==
  Xdot : Inport
  Constant : Constant  Value=Xo
  Integrator : Integrator  InitialConditionSource=external
  X : Outport
  wires:
  Integrator/1 -> X/1
  Xdot/1 -> Integrator/1
  Constant/1 -> Integrator/2

== system Lib_EMTAT/Loop Blocks/Outer Loop Time Step Delay ==
  W(t) : Inport
  Unit Delay : UnitDelay  InitialCondition=Wo  SampleTime=-1  HasFrameUpgradeWarning=on
  W(t-1) : Outport
  wires:
  W(t)/1 -> Unit Delay/1
  Unit Delay/1 -> W(t-1)/1

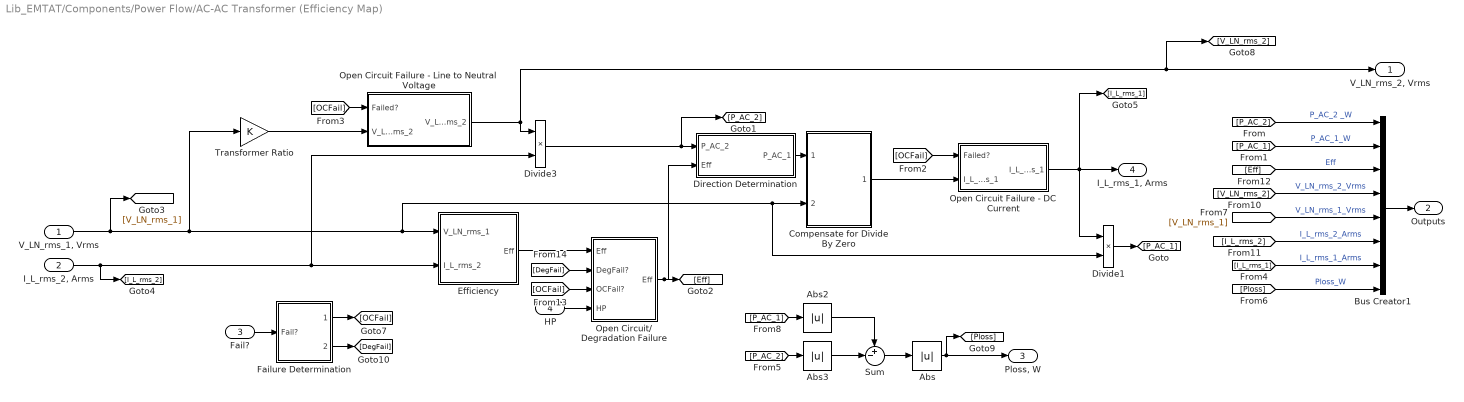
== system Lib_EMTAT/Components/Power Flow/AC-AC Transformer (Efficiency Map) ==
  "V_LN_rms_1, Vrms" : Inport
  "I_L_rms_2, Arms" : Inport  Port=2
  Fail? : Inport  Port=3
  HP : Inport  Port=4
  Abs : Abs  SaturateOnIntegerOverflow=off
  Abs2 : Abs  SaturateOnIntegerOverflow=off
  Abs3 : Abs  SaturateOnIntegerOverflow=off
  Bus Creator1 : BusCreator  Inputs=8
  Compensate for Divide By Zero : Subsystem
  Direction Determination : Subsystem
  Divide1 : Product  Inputs=**
  Divide3 : Product  Inputs=**
  Efficiency : Subsystem
  Failure Determination : Subsystem
  Open Circuit Failure - DC Current : Subsystem
  Open Circuit Failure - Line to Neutral Voltage : Subsystem
  Open Circuit/ Degradation Failure : Subsystem
  Sum : Sum  Inputs=+-|
  Transformer Ratio : Gain  Gain=K
  "V_LN_rms_2, Vrms" : Outport
  Outputs : Outport  Port=2
  "Ploss, W" : Outport  Port=3
  "I_L_rms_1, Arms" : Outport  Port=4
  wires:
  [DegFail] -> Open Circuit/ Degradation Failure/2(DegFail?)
  [OCFail] -> Open Circuit/ Degradation Failure/3(OCFail?)
  HP/1 -> Open Circuit/ Degradation Failure/4(HP)
  Fail?/1 -> Failure Determination/1(Fail?)
  Failure Determination/1(OCFail) -> [OCFail]
  Failure Determination/2(DegFail) -> [DegFail]
  Efficiency/1(Eff) -> Open Circuit/ Degradation Failure/1(Eff)
  Open Circuit Failure - Line to Neutral Voltage/1("V_LN_rms_2 ") -> Divide3/1, [V_LN_rms_2], "V_LN_rms_2, Vrms"/1
  [OCFail] -> Open Circuit Failure - Line to Neutral Voltage/1(Failed?)
  Transformer Ratio/1 -> Open Circuit Failure - Line to Neutral Voltage/2(V_LN_rms_2)
  [OCFail] -> Open Circuit Failure - DC Current/1(Failed?)
  [Eff] -> Bus Creator1/3  "Eff"
  [I_L_rms_2] -> Bus Creator1/6  "I_L_rms_2_Arms"
  [Ploss] -> Bus Creator1/8  "Ploss_W"
  [I_L_rms_1] -> Bus Creator1/7  "I_L_rms_1_Arms"
  [V_LN_rms_1] -> Bus Creator1/5  "V_LN_rms_1_Vrms"
  [V_LN_rms_2] -> Bus Creator1/4  "V_LN_rms_2_Vrms"
  "I_L_rms_2, Arms"/1 -> [I_L_rms_2], Divide3/2, Efficiency/2(I_L_rms_2)
  Divide3/1 -> Direction Determination/1(P_AC_2), [P_AC_2]
  Open Circuit Failure - DC Current/1("I_L_rms_1 ") -> [I_L_rms_1], "I_L_rms_1, Arms"/1, Divide1/1
  Open Circuit/ Degradation Failure/1("Eff ") -> Direction Determination/2(Eff), [Eff]
  [P_AC_1] -> Bus Creator1/2  "P_AC_1_W"
  [P_AC_2] -> Bus Creator1/1  "P_AC_2 _W"
  Bus Creator1/1 -> Outputs/1
  Direction Determination/1(P_AC_1) -> Compensate for Divide By Zero/1(P_AC_1)
  Divide1/1 -> [P_AC_1]
  "V_LN_rms_1, Vrms"/1 -> Transformer Ratio/1, Divide1/2, Compensate for Divide By Zero/2(V_LN_rms_1), Efficiency/1(V_LN_rms_1), [V_LN_rms_1]
  Compensate for Divide By Zero/1(I_L_rms_1) -> Open Circuit Failure - DC Current/2(I_L_rms_1)
  Abs2/1 -> Sum/1
  Sum/1 -> Abs/1
  [P_AC_1] -> Abs2/1
  Abs3/1 -> Sum/2
  Abs/1 -> "Ploss, W"/1, [Ploss]
  [P_AC_2] -> Abs3/1

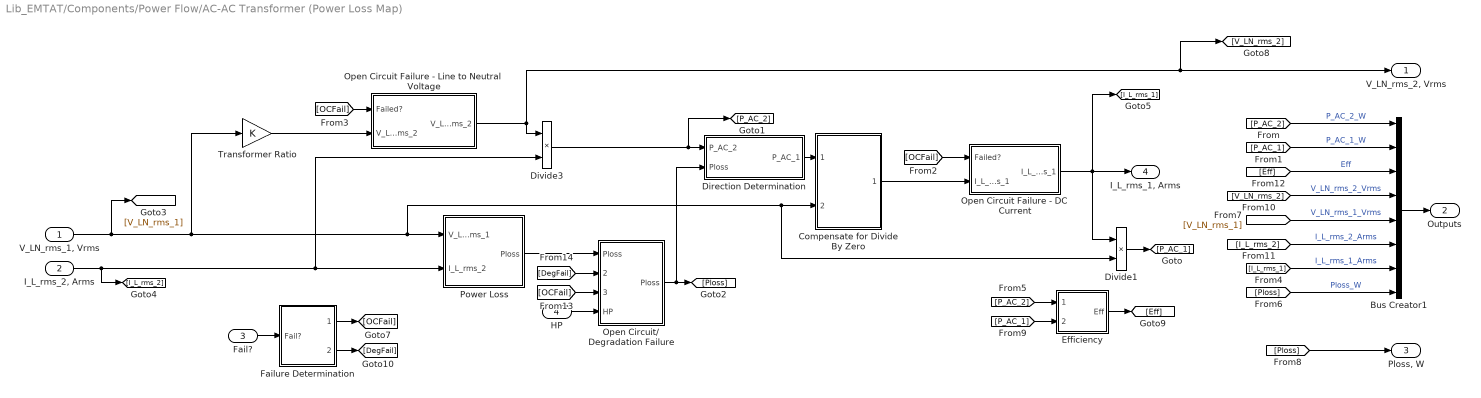
== system Lib_EMTAT/Components/Power Flow/AC-AC Transformer (Power Loss Map) ==
  "V_LN_rms_1, Vrms" : Inport
  "I_L_rms_2, Arms" : Inport  Port=2
  Fail? : Inport  Port=3
  HP : Inport  Port=4
  Bus Creator1 : BusCreator  Inputs=8
  Compensate for Divide By Zero : Subsystem
  Direction Determination : Subsystem
  Divide1 : Product  Inputs=**
  Divide3 : Product  Inputs=**
  Efficiency : Subsystem
  Failure Determination : Subsystem
  Open Circuit Failure - DC Current : Subsystem
  Open Circuit Failure - Line to Neutral Voltage : Subsystem
  Open Circuit/ Degradation Failure : Subsystem
  Power Loss : Subsystem
  Transformer Ratio : Gain  Gain=K
  "V_LN_rms_2, Vrms" : Outport
  Outputs : Outport  Port=2
  "Ploss, W" : Outport  Port=3
  "I_L_rms_1, Arms" : Outport  Port=4
  wires:
  Compensate for Divide By Zero/1(I_L_rms_1) -> Open Circuit Failure - DC Current/2(I_L_rms_1)
  "V_LN_rms_1, Vrms"/1 -> [V_LN_rms_1], Power Loss/1(V_LN_rms_1), Compensate for Divide By Zero/2(V_LN_rms_1), Divide1/2, Transformer Ratio/1
  Divide1/1 -> [P_AC_1]
  Direction Determination/1(P_AC_1) -> Compensate for Divide By Zero/1(P_AC_1)
  Bus Creator1/1 -> Outputs/1
  [P_AC_2] -> Bus Creator1/1  "P_AC_2_W"
  [P_AC_1] -> Bus Creator1/2  "P_AC_1_W"
  Open Circuit/ Degradation Failure/1("Ploss ") -> Direction Determination/2(Ploss), [Ploss]
  Open Circuit Failure - DC Current/1("I_L_rms_1 ") -> Divide1/1, "I_L_rms_1, Arms"/1, [I_L_rms_1]
  Divide3/1 -> Direction Determination/1(P_AC_2), [P_AC_2]
  [Ploss] -> "Ploss, W"/1
  "I_L_rms_2, Arms"/1 -> Power Loss/2(I_L_rms_2), Divide3/2, [I_L_rms_2]
  [V_LN_rms_2] -> Bus Creator1/4  "V_LN_rms_2_Vrms"
  [V_LN_rms_1] -> Bus Creator1/5  "V_LN_rms_1_Vrms"
  [I_L_rms_1] -> Bus Creator1/7  "I_L_rms_1_Arms"
  [Ploss] -> Bus Creator1/8  "Ploss_W"
  [I_L_rms_2] -> Bus Creator1/6  "I_L_rms_2_Arms"
  [P_AC_1] -> Efficiency/2(P_AC_1)
  [P_AC_2] -> Efficiency/1(P_AC_2)
  Efficiency/1(Eff) -> [Eff]
  [Eff] -> Bus Creator1/3  "Eff"
  [OCFail] -> Open Circuit Failure - DC Current/1(Failed?)
  Transformer Ratio/1 -> Open Circuit Failure - Line to Neutral Voltage/2(V_LN_rms_2)
  [OCFail] -> Open Circuit Failure - Line to Neutral Voltage/1(Failed?)
  Open Circuit Failure - Line to Neutral Voltage/1("V_LN_rms_2 ") -> "V_LN_rms_2, Vrms"/1, [V_LN_rms_2], Divide3/1
  Power Loss/1(Ploss) -> Open Circuit/ Degradation Failure/1(Ploss)
  Failure Determination/2(DegFail) -> [DegFail]
  Failure Determination/1(OCFail) -> [OCFail]
  Fail?/1 -> Failure Determination/1(Fail?)
  HP/1 -> Open Circuit/ Degradation Failure/4(HP)
  [OCFail] -> Open Circuit/ Degradation Failure/3(OCFail?)
  [DegFail] -> Open Circuit/ Degradation Failure/2(DegFail?)

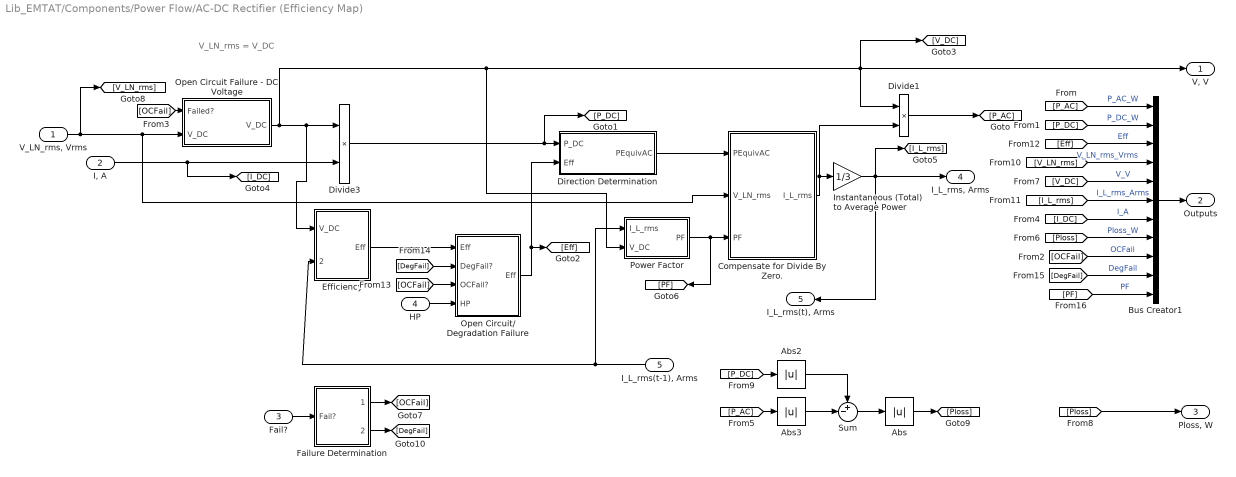
== system Lib_EMTAT/Components/Power Flow/AC-DC Rectifier (Efficiency Map) ==
  note: V_LN_rms = V_DC
  "V_LN_rms, Vrms" : Inport
  "I, A" : Inport  Port=2
  Fail? : Inport  Port=3
  HP : Inport  Port=4
  "I_L_rms(t-1), Arms" : Inport  Port=5
  Abs : Abs  SaturateOnIntegerOverflow=off
  Abs2 : Abs  SaturateOnIntegerOverflow=off
  Abs3 : Abs  SaturateOnIntegerOverflow=off
  Bus Creator1 : BusCreator  Inputs=11
  Compensate for Divide By Zero. : Subsystem
  Direction Determination : Subsystem
  Divide1 : Product  Inputs=**
  Divide3 : Product  Inputs=**
  Efficiency : Subsystem
  Failure Determination : Subsystem
  Instantaneous (Total) to Average Power : Gain  Gain=1/3
  Open Circuit Failure - DC Voltage : Subsystem
  Open Circuit/ Degradation Failure : Subsystem
  Power Factor : Subsystem
  Sum : Sum  Inputs=+-|
  "V, V " : Outport
  Outputs : Outport  Port=2
  "Ploss, W" : Outport  Port=3
  "I_L_rms, Arms" : Outport  Port=4
  "I_L_rms(t), Arms" : Outport  Port=5
  wires:
  Divide1/1 -> [P_AC]
  "I, A"/1 -> [I_DC], Divide3/2
  Compensate for Divide By Zero./1(I_L_rms) -> Divide1/2, Instantaneous (Total) to Average Power/1
  [Eff] -> Bus Creator1/3  "Eff"
  [I_L_rms] -> Bus Creator1/6  "I_L_rms_Arms"
  [Ploss] -> Bus Creator1/8  "Ploss_W"
  [I_DC] -> Bus Creator1/7  "I_A"
  [V_DC] -> Bus Creator1/5  "V_V"
  [V_LN_rms] -> Bus Creator1/4  "V_LN_rms_Vrms"
  [Ploss] -> "Ploss, W"/1
  Divide3/1 -> Direction Determination/1(P_DC), [P_DC]
  Open Circuit/ Degradation Failure/1("Eff ") -> Direction Determination/2(Eff), [Eff]
  [P_DC] -> Bus Creator1/2  "P_DC_W"
  [P_AC] -> Bus Creator1/1  "P_AC_W"
  Bus Creator1/1 -> Outputs/1
  Direction Determination/1(PEquivAC) -> Compensate for Divide By Zero./1(PEquivAC)
  "I_L_rms(t-1), Arms"/1 -> Efficiency/2(I_L_rms), Power Factor/1(I_L_rms)
  Instantaneous (Total) to Average Power/1 -> [I_L_rms], "I_L_rms(t), Arms"/1, "I_L_rms, Arms"/1
  [OCFail] -> Open Circuit Failure - DC Voltage/1(Failed?)
  "V_LN_rms, Vrms"/1 -> [V_LN_rms], Compensate for Divide By Zero./2(V_LN_rms), Open Circuit Failure - DC Voltage/2(V_DC)
  [OCFail] -> Open Circuit/ Degradation Failure/3(OCFail?)
  [DegFail] -> Open Circuit/ Degradation Failure/2(DegFail?)
  HP/1 -> Open Circuit/ Degradation Failure/4(HP)
  Efficiency/1(Eff) -> Open Circuit/ Degradation Failure/1(Eff)
  Fail?/1 -> Failure Determination/1(Fail?)
  Failure Determination/2(DegFail) -> [DegFail]
  Failure Determination/1(OCFail) -> [OCFail]
  Open Circuit Failure - DC Voltage/1("V_DC ") -> Efficiency/1(V_DC), Divide3/1, "V, V "/1, Divide1/1, [V_DC], Power Factor/2(V_DC)
  [P_AC] -> Abs3/1
  Abs3/1 -> Sum/2
  [P_DC] -> Abs2/1
  Sum/1 -> Abs/1
  Abs2/1 -> Sum/1
  Abs/1 -> [Ploss]
  Power Factor/1(PF) -> [PF], Compensate for Divide By Zero./3(PF)
  [OCFail] -> Bus Creator1/9  "OCFail"
  [DegFail] -> Bus Creator1/10  "DegFail"
  [PF] -> Bus Creator1/11  "PF"

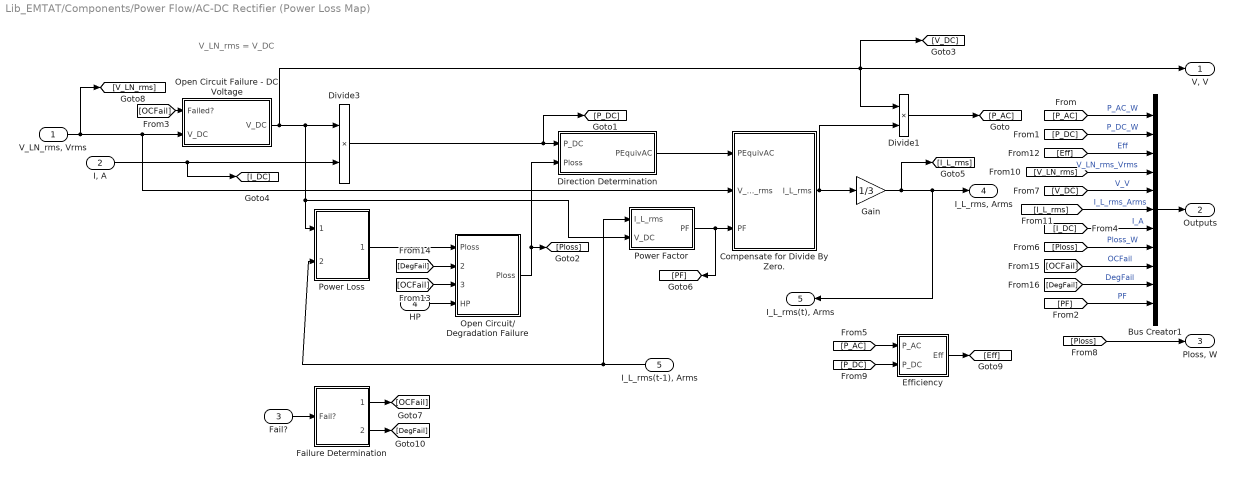
== system Lib_EMTAT/Components/Power Flow/AC-DC Rectifier (Power Loss Map) ==
  note: V_LN_rms = V_DC
  "V_LN_rms, Vrms" : Inport
  "I, A" : Inport  Port=2
  Fail? : Inport  Port=3
  HP : Inport  Port=4
  "I_L_rms(t-1), Arms" : Inport  Port=5
  Bus Creator1 : BusCreator  Inputs=11
  Compensate for Divide By Zero. : Subsystem
  Direction Determination : Subsystem
  Divide1 : Product  Inputs=**
  Divide3 : Product  Inputs=**
  Efficiency : Subsystem
  Failure Determination : Subsystem
  Gain : Gain  Gain=1/3
  Open Circuit Failure - DC Voltage : Subsystem
  Open Circuit/ Degradation Failure : Subsystem
  Power Factor : Subsystem
  Power Loss : Subsystem
  "V, V " : Outport
  Outputs : Outport  Port=2
  "Ploss, W" : Outport  Port=3
  "I_L_rms, Arms" : Outport  Port=4
  "I_L_rms(t), Arms" : Outport  Port=5
  wires:
  Open Circuit Failure - DC Voltage/1("V_DC ") -> [V_DC], Divide1/1, "V, V "/1, Divide3/1, Power Factor/2(V_DC), Power Loss/1(V_DC)
  Failure Determination/1(OCFail) -> [OCFail]
  Failure Determination/2(DegFail) -> [DegFail]
  Fail?/1 -> Failure Determination/1(Fail?)
  Power Loss/1(Ploss) -> Open Circuit/ Degradation Failure/1(Ploss)
  HP/1 -> Open Circuit/ Degradation Failure/4(HP)
  [DegFail] -> Open Circuit/ Degradation Failure/2(DegFail?)
  [OCFail] -> Open Circuit/ Degradation Failure/3(OCFail?)
  "V_LN_rms, Vrms"/1 -> Open Circuit Failure - DC Voltage/2(V_DC), Compensate for Divide By Zero./2(V_LN_rms), [V_LN_rms]
  [OCFail] -> Open Circuit Failure - DC Voltage/1(Failed?)
  Gain/1 -> "I_L_rms, Arms"/1, "I_L_rms(t), Arms"/1, [I_L_rms]
  "I_L_rms(t-1), Arms"/1 -> Power Factor/1(I_L_rms), Power Loss/2(I_L_rms)
  Direction Determination/1(PEquivAC) -> Compensate for Divide By Zero./1(PEquivAC)
  Bus Creator1/1 -> Outputs/1
  [P_AC] -> Bus Creator1/1  "P_AC_W"
  [P_DC] -> Bus Creator1/2  "P_DC_W"
  Open Circuit/ Degradation Failure/1("Ploss ") -> [Ploss], Direction Determination/2(Ploss)
  Divide3/1 -> [P_DC], Direction Determination/1(P_DC)
  [Ploss] -> "Ploss, W"/1
  [V_LN_rms] -> Bus Creator1/4  "V_LN_rms_Vrms"
  [V_DC] -> Bus Creator1/5  "V_V"
  [I_DC] -> Bus Creator1/7  "I_A"
  [Ploss] -> Bus Creator1/8  "Ploss_W"
  [I_L_rms] -> Bus Creator1/6  "I_L_rms_Arms"
  [P_DC] -> Efficiency/2(P_DC)
  [P_AC] -> Efficiency/1(P_AC)
  Efficiency/1(Eff) -> [Eff]
  [Eff] -> Bus Creator1/3  "Eff"
  Compensate for Divide By Zero./1(I_L_rms) -> Divide1/2, Gain/1
  "I, A"/1 -> Divide3/2, [I_DC]
  Divide1/1 -> [P_AC]
  Power Factor/1(PF) -> [PF], Compensate for Divide By Zero./3(PF)
  [PF] -> Bus Creator1/11  "PF"
  [OCFail] -> Bus Creator1/9  "OCFail"
  [DegFail] -> Bus Creator1/10  "DegFail"
